simulink library "RWSW"  (Simulink 9.2)
settings: Solver=ode45  StartTime=0.0  StopTime=10.0  RelTol=1e-3  EnableMultiTasking=on
libraries: ACT x1, DYN x1, SEN x1
settings Model: Creator=alger  LastModifiedBy=alger

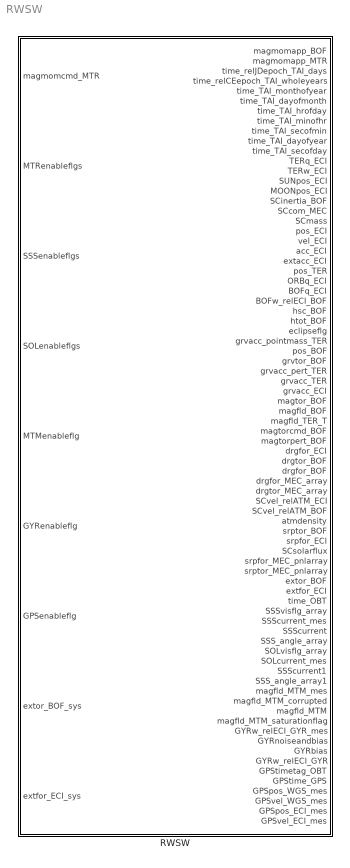
== system RWSW ==
  RWSW : Subsystem

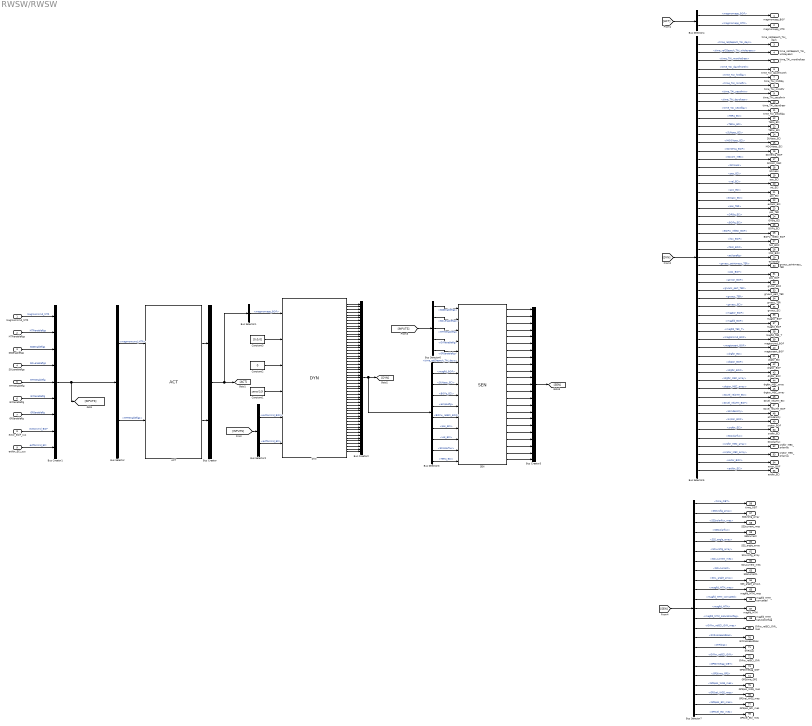
== system RWSW/RWSW ==
  magmomcmd_MTR : Inport  PortDimensions=10
  MTRenableflgs : Inport  Port=2  PortDimensions=10
  SSSenableflgs : Inport  Port=3  PortDimensions=10
  SOLenableflgs : Inport  Port=4  PortDimensions=10
  MTMenableflg : Inport  Port=5  PortDimensions=1
  GYRenableflg : Inport  Port=6  PortDimensions=1
  GPSenableflg : Inport  Port=7  PortDimensions=1
  extor_BOF_sys : Inport  Port=8  PortDimensions=3
  extfor_ECI_sys : Inport  Port=9  PortDimensions=3
  ACT : ACT/ACT  SystemSampleTime=-1
  Bus Creator : BusCreator  Inputs=2
  Bus Creator1 : BusCreator  Inputs=9
  Bus Creator2 : BusCreator  Inputs=55
  Bus Creator3 : BusCreator  Inputs=23
  Bus Selector : BusSelector  OutputSignals=magmomcmd_MTR,MTRenableflgs
  Bus Selector1 : BusSelector  OutputSignals=magmomapp_BOF
  Bus Selector2 : BusSelector  OutputSignals=exttorcmd_BOF,extforcmd_ECI
  Bus Selector3 : BusSelector  OutputSignals=time_relJDepoch_TAI_days,magfld_BOF,SUNpos_ECI,BOFq_ECI,eclipseflg,BOFw_relECI_BOF,pos_ECI,vel_ECI,SCsolarflux,TERq_ECI
  Bus Selector4 : BusSelector  OutputSignals=magmomapp_BOF,magmomapp_MTR
  Bus Selector5 : BusSelector  OutputSignals=time_relJDepoch_TAI_days,time_relCEepoch_TAI_wholeyears,time_TAI_monthofyear,time_TAI_dayofmonth,time_TAI_hrofday,time_TAI_minofhr,time_TAI_secofmin,time_TAI_dayofyear,time_TAI_secofday,TERq_ECI,TERw_ECI,SUNpos_ECI,MOONpos_ECI,SCinertia_BOF,SCcom_MEC,SCmass,pos_ECI,vel_ECI,acc_ECI,extacc_ECI,pos_TER,ORBq_ECI,BOFq_ECI,BOFw_relECI_BOF,hsc_BOF,htot_BOF,eclipseflg,grvacc_pointmass_TER,pos_BOF,grvtor_BOF,grvacc_pert_TER,grvacc_TER,grvacc_ECI,magtor_BOF,magfld_BOF,magfld_TER_T,magtorcmd_BOF,magtorpert_BOF,drgfor_ECI,drgtor_BOF,drgfor_BOF,drgfor_MEC_array,drgtor_MEC_array,SCvel_relATM_ECI,SCvel_relATM_BOF,atmdensity,srptor_BOF,srpfor_ECI,SCsolarflux,srpfor_MEC_array,srptor_MEC_array,extor_BOF,extfor_ECI
  Bus Selector6 : BusSelector  OutputSignals=SSSenableflgs,SOLenableflgs,MTMenableflg,GYRenableflg,GPSenableflg
  Bus Selector7 : BusSelector  OutputSignals=time_OBT,SSSvisflg_array,SSSsolarflux_mes,SSSsolarflux,SSS_angle_array,SOLvisflg_array,SOLcurrent_mes,SOLcurrent,SOL_angle_array,magfld_MTM_mes,magfld_MTM_corrupted,magfld_MTM,magfld_MTM_saturationflag,GYRw_relECI_GYR_mes,GYRnoiseandbias,GYRbias,GYRw_relECI_GYR,GPStimetag_OBT,GPStime_GPS,GPSpos_WGS_mes,GPSvel_WGS_mes,GPSpos_ECI_mes,GPSvel_ECI_mes
  Constant1 : Constant  Value=zeros(3,3)
  Constant2 : Constant  Value=0
  Constant3 : Constant  Value=[0;0;0]
  DYN : DYN/DYN  SystemSampleTime=-1
  SEN : SEN/SEN  SystemSampleTime=-1
  "magmomapp_BOF " : Outport
  magmomapp_MTR : Outport  Port=2
  time_relJDepoch_TAI_days : Outport  Port=3
  time_relCEepoch_TAI_wholeyears : Outport  Port=4
  time_TAI_monthofyear : Outport  Port=5
  time_TAI_dayofmonth : Outport  Port=6
  time_TAI_hrofday : Outport  Port=7
  time_TAI_minofhr : Outport  Port=8
  time_TAI_secofmin : Outport  Port=9
  time_TAI_dayofyear : Outport  Port=10
  time_TAI_secofday : Outport  Port=11
  TERq_ECI : Outport  Port=12
  TERw_ECI : Outport  Port=13
  SUNpos_ECI : Outport  Port=14
  MOONpos_ECI : Outport  Port=15
  SCinertia_BOF : Outport  Port=16
  SCcom_MEC : Outport  Port=17
  SCmass : Outport  Port=18
  pos_ECI : Outport  Port=19
  vel_ECI : Outport  Port=20
  acc_ECI : Outport  Port=21
  extacc_ECI : Outport  Port=22
  pos_TER : Outport  Port=23
  ORBq_ECI : Outport  Port=24
  BOFq_ECI : Outport  Port=25
  BOFw_relECI_BOF : Outport  Port=26
  hsc_BOF : Outport  Port=27
  htot_BOF : Outport  Port=28
  eclipseflg : Outport  Port=29
  grvacc_pointmass_TER : Outport  Port=30
  pos_BOF : Outport  Port=31
  grvtor_BOF : Outport  Port=32
  grvacc_pert_TER : Outport  Port=33
  grvacc_TER : Outport  Port=34
  grvacc_ECI : Outport  Port=35
  magtor_BOF : Outport  Port=36
  magfld_BOF : Outport  Port=37
  magfld_TER_T : Outport  Port=38
  magtorcmd_BOF : Outport  Port=39
  magtorpert_BOF : Outport  Port=40
  drgfor_ECI : Outport  Port=41
  drgtor_BOF : Outport  Port=42
  drgfor_BOF : Outport  Port=43
  drgfor_MEC_array : Outport  Port=44
  drgtor_MEC_array : Outport  Port=45
  SCvel_relATM_ECI : Outport  Port=46
  SCvel_relATM_BOF : Outport  Port=47
  atmdensity : Outport  Port=48
  srptor_BOF : Outport  Port=49  PortDimensions=3
  srpfor_ECI : Outport  Port=50  PortDimensions=3
  SCsolarflux : Outport  Port=51
  srpfor_MEC_pnlarray : Outport  Port=52
  srptor_MEC_pnlarray : Outport  Port=53
  extor_BOF : Outport  Port=54
  extfor_ECI : Outport  Port=55
  time_OBT : Outport  Port=56
  SSSvisflg_array : Outport  Port=57
  SSScurrent_mes : Outport  Port=58
  SSScurrent : Outport  Port=59
  SSS_angle_array : Outport  Port=60
  SOLvisflg_array : Outport  Port=61
  SOLcurrent_mes : Outport  Port=62
  SSScurrent1 : Outport  Port=63
  SSS_angle_array1 : Outport  Port=64
  magfld_MTM_mes : Outport  Port=65
  magfld_MTM_corrupted : Outport  Port=66
  magfld_MTM : Outport  Port=67
  magfld_MTM_saturationflag : Outport  Port=68
  GYRw_relECI_GYR_mes : Outport  Port=69  PortDimensions=3
  GYRnoiseandbias : Outport  Port=70  PortDimensions=3
  GYRbias : Outport  Port=71  PortDimensions=3
  GYRw_relECI_GYR : Outport  Port=72  PortDimensions=3
  GPStimetag_OBT : Outport  Port=73
  GPStime_GPS : Outport  Port=74
  GPSpos_WGS_mes : Outport  Port=75
  GPSvel_WGS_mes : Outport  Port=76
  GPSpos_ECI_mes : Outport  Port=77
  GPSvel_ECI_mes : Outport  Port=78
  wires:
  magmomcmd_MTR/1 -> Bus Creator1/1  "magmomcmd_MTR"
  Constant1/1 -> DYN/4
  ACT/1 -> Bus Creator/1
  ACT/2 -> Bus Creator/2
  extor_BOF_sys/1 -> Bus Creator1/8  "exttorcmd_BOF"
  extfor_ECI_sys/1 -> Bus Creator1/9  "extforcmd_ECI"
  Bus Creator1/1 -> Bus Selector/1, [INPUTS]
  Bus Selector/1 -> ACT/1  "<magmomcmd_MTR>"
  Bus Creator/1 -> Bus Selector1/1, [ACT]
  Constant2/1 -> DYN/3
  Constant3/1 -> DYN/2
  Bus Selector1/1 -> DYN/1  "<magmomapp_BOF>"
  [INPUTS] -> Bus Selector2/1
  Bus Selector2/1 -> DYN/5  "<exttorcmd_BOF>"
  Bus Selector2/2 -> DYN/6  "<extforcmd_ECI>"
  DYN/31 -> Bus Creator2/31
  DYN/10 -> Bus Creator2/10
  DYN/23 -> Bus Creator2/23
  DYN/27 -> Bus Creator2/27
  DYN/3 -> Bus Creator2/3
  DYN/46 -> Bus Creator2/46
  DYN/47 -> Bus Creator2/47
  DYN/22 -> Bus Creator2/22
  DYN/35 -> Bus Creator2/35
  DYN/37 -> Bus Creator2/37
  DYN/36 -> Bus Creator2/36
  DYN/2 -> Bus Creator2/2
  DYN/38 -> Bus Creator2/38
  DYN/40 -> Bus Creator2/40
  DYN/12 -> Bus Creator2/12
  DYN/24 -> Bus Creator2/24
  DYN/11 -> Bus Creator2/11
  DYN/42 -> Bus Creator2/42
  DYN/48 -> Bus Creator2/48
  DYN/26 -> Bus Creator2/26
  DYN/5 -> Bus Creator2/5
  DYN/8 -> Bus Creator2/8
  DYN/7 -> Bus Creator2/7
  DYN/13 -> Bus Creator2/13
  DYN/14 -> Bus Creator2/14
  DYN/16 -> Bus Creator2/16
  DYN/34 -> Bus Creator2/34
  DYN/41 -> Bus Creator2/41
  DYN/43 -> Bus Creator2/43
  DYN/6 -> Bus Creator2/6
  DYN/15 -> Bus Creator2/15
  DYN/49 -> Bus Creator2/49
  DYN/9 -> Bus Creator2/9
  DYN/50 -> Bus Creator2/50
  DYN/19 -> Bus Creator2/19
  DYN/4 -> Bus Creator2/4
  DYN/1 -> Bus Creator2/1
  DYN/18 -> Bus Creator2/18
  DYN/25 -> Bus Creator2/25
  DYN/29 -> Bus Creator2/29
  DYN/30 -> Bus Creator2/30
  DYN/20 -> Bus Creator2/20
  DYN/32 -> Bus Creator2/32
  DYN/28 -> Bus Creator2/28
  DYN/52 -> Bus Creator2/52
  DYN/21 -> Bus Creator2/21
  DYN/33 -> Bus Creator2/33
  DYN/39 -> Bus Creator2/39
  DYN/53 -> Bus Creator2/53
  DYN/17 -> Bus Creator2/17
  DYN/51 -> Bus Creator2/51
  DYN/44 -> Bus Creator2/44
  DYN/45 -> Bus Creator2/45
  Bus Creator2/1 -> Bus Selector3/1, [DYN]
  [ACT] -> Bus Selector4/1
  Bus Selector4/1 -> "magmomapp_BOF "/1  "<magmomapp_BOF>"
  Bus Selector4/2 -> magmomapp_MTR/1  "<magmomapp_MTR>"
  [DYN] -> Bus Selector5/1
  Bus Selector5/10 -> TERq_ECI/1  "<TERq_ECI>"
  Bus Selector5/11 -> TERw_ECI/1  "<TERw_ECI>"
  Bus Selector5/13 -> MOONpos_ECI/1  "<MOONpos_ECI>"
  Bus Selector5/12 -> SUNpos_ECI/1  "<SUNpos_ECI>"
  Bus Selector5/16 -> SCmass/1  "<SCmass>"
  Bus Selector5/15 -> SCcom_MEC/1  "<SCcom_MEC>"
  Bus Selector5/14 -> SCinertia_BOF/1  "<SCinertia_BOF>"
  Bus Selector5/22 -> ORBq_ECI/1  "<ORBq_ECI>"
  Bus Selector5/21 -> pos_TER/1  "<pos_TER>"
  Bus Selector5/19 -> acc_ECI/1  "<acc_ECI>"
  Bus Selector5/18 -> vel_ECI/1  "<vel_ECI>"
  Bus Selector5/17 -> pos_ECI/1  "<pos_ECI>"
  Bus Selector5/20 -> extacc_ECI/1  "<extacc_ECI>"
  Bus Selector5/2 -> time_relCEepoch_TAI_wholeyears/1  "<time_relCEepoch_TAI_wholeyears>"
  Bus Selector5/3 -> time_TAI_monthofyear/1  "<time_TAI_monthofyear>"
  Bus Selector5/6 -> time_TAI_minofhr/1  "<time_TAI_minofhr>"
  Bus Selector5/9 -> time_TAI_secofday/1  "<time_TAI_secofday>"
  Bus Selector5/1 -> time_relJDepoch_TAI_days/1  "<time_relJDepoch_TAI_days>"
  Bus Selector5/7 -> time_TAI_secofmin/1  "<time_TAI_secofmin>"
  Bus Selector5/4 -> time_TAI_dayofmonth/1  "<time_TAI_dayofmonth>"
  Bus Selector5/5 -> time_TAI_hrofday/1  "<time_TAI_hrofday>"
  Bus Selector5/8 -> time_TAI_dayofyear/1  "<time_TAI_dayofyear>"
  Bus Selector5/23 -> BOFq_ECI/1  "<BOFq_ECI>"
  Bus Selector5/24 -> BOFw_relECI_BOF/1  "<BOFw_relECI_BOF>"
  Bus Selector5/25 -> hsc_BOF/1  "<hsc_BOF>"
  Bus Selector5/26 -> htot_BOF/1  "<htot_BOF>"
  Bus Selector5/27 -> eclipseflg/1  "<eclipseflg>"
  Bus Selector5/28 -> grvacc_pointmass_TER/1  "<grvacc_pointmass_TER>"
  Bus Selector5/29 -> pos_BOF/1  "<pos_BOF>"
  Bus Selector5/30 -> grvtor_BOF/1  "<grvtor_BOF>"
  Bus Selector5/31 -> grvacc_pert_TER/1  "<grvacc_pert_TER>"
  Bus Selector5/32 -> grvacc_TER/1  "<grvacc_TER>"
  Bus Selector5/33 -> grvacc_ECI/1  "<grvacc_ECI>"
  Bus Selector5/34 -> magtor_BOF/1  "<magtor_BOF>"
  Bus Selector5/36 -> magfld_TER_T/1  "<magfld_TER_T>"
  Bus Selector5/38 -> magtorpert_BOF/1  "<magtorpert_BOF>"
  Bus Selector5/35 -> magfld_BOF/1  "<magfld_BOF>"
  Bus Selector5/37 -> magtorcmd_BOF/1  "<magtorcmd_BOF>"
  Bus Selector5/44 -> SCvel_relATM_ECI/1  "<SCvel_relATM_ECI>"
  Bus Selector5/39 -> drgfor_ECI/1  "<drgfor_ECI>"
  Bus Selector5/42 -> drgfor_MEC_array/1  "<drgfor_MEC_array>"
  Bus Selector5/43 -> drgtor_MEC_array/1  "<drgtor_MEC_array>"
  Bus Selector5/45 -> SCvel_relATM_BOF/1  "<SCvel_relATM_BOF>"
  Bus Selector5/46 -> atmdensity/1  "<atmdensity>"
  Bus Selector5/40 -> drgtor_BOF/1  "<drgtor_BOF>"
  Bus Selector5/41 -> drgfor_BOF/1  "<drgfor_BOF>"
  Bus Selector5/47 -> srptor_BOF/1  "<srptor_BOF>"
  Bus Selector5/48 -> srpfor_ECI/1  "<srpfor_ECI>"
  Bus Selector5/49 -> SCsolarflux/1  "<SCsolarflux>"
  Bus Selector5/50 -> srpfor_MEC_pnlarray/1  "<srpfor_MEC_array>"
  Bus Selector5/51 -> srptor_MEC_pnlarray/1  "<srptor_MEC_array>"
  Bus Selector5/52 -> extor_BOF/1  "<extor_BOF>"
  Bus Selector5/53 -> extfor_ECI/1  "<extfor_ECI>"
  MTRenableflgs/1 -> Bus Creator1/2  "MTRenableflgs"
  Bus Selector/2 -> ACT/2  "<MTRenableflgs>"
  [INPUTS] -> Bus Selector6/1
  MTMenableflg/1 -> Bus Creator1/5  "MTMenableflg"
  SSSenableflgs/1 -> Bus Creator1/3  "SSSenableflgs"
  GYRenableflg/1 -> Bus Creator1/6  "GYRenableflg"
  GPSenableflg/1 -> Bus Creator1/7  "GPSenableflg"
  Bus Creator3/1 -> [SEN]
  [SEN] -> Bus Selector7/1
  SOLenableflgs/1 -> Bus Creator1/4  "SOLenableflgs"
  Bus Selector6/2 -> SEN/2  "<SOLenableflgs>"
  Bus Selector6/4 -> SEN/4  "<GYRenableflg>"
  Bus Selector6/1 -> SEN/1  "<SSSenableflgs>"
  Bus Selector6/3 -> SEN/3  "<MTMenableflg>"
  Bus Selector6/5 -> SEN/5  "<GPSenableflg>"
  Bus Selector3/6 -> SEN/11  "<BOFw_relECI_BOF>"
  Bus Selector3/5 -> SEN/10  "<eclipseflg>"
  Bus Selector3/7 -> SEN/12  "<pos_ECI>"
  Bus Selector3/4 -> SEN/9  "<BOFq_ECI>"
  Bus Selector3/8 -> SEN/13  "<vel_ECI>"
  Bus Selector3/9 -> SEN/14  "<SCsolarflux>"
  Bus Selector3/3 -> SEN/8  "<SUNpos_ECI>"
  Bus Selector3/2 -> SEN/7  "<magfld_BOF>"
  Bus Selector3/1 -> SEN/6  "<time_relJDepoch_TAI_days>"
  SEN/1 -> Bus Creator3/1
  SEN/5 -> Bus Creator3/5
  SEN/17 -> Bus Creator3/17
  SEN/18 -> Bus Creator3/18
  SEN/20 -> Bus Creator3/20
  SEN/21 -> Bus Creator3/21
  SEN/22 -> Bus Creator3/22
  SEN/4 -> Bus Creator3/4
  SEN/8 -> Bus Creator3/8
  SEN/10 -> Bus Creator3/10
  SEN/19 -> Bus Creator3/19
  SEN/9 -> Bus Creator3/9
  SEN/11 -> Bus Creator3/11
  SEN/2 -> Bus Creator3/2
  SEN/12 -> Bus Creator3/12
  SEN/6 -> Bus Creator3/6
  SEN/15 -> Bus Creator3/15
  SEN/13 -> Bus Creator3/13
  SEN/7 -> Bus Creator3/7
  SEN/3 -> Bus Creator3/3
  SEN/14 -> Bus Creator3/14
  SEN/16 -> Bus Creator3/16
  Bus Selector7/1 -> time_OBT/1  "<time_OBT>"
  Bus Selector7/2 -> SSSvisflg_array/1  "<SSSvisflg_array>"
  Bus Selector7/3 -> SSScurrent_mes/1  "<SSSsolarflux_mes>"
  Bus Selector7/4 -> SSScurrent/1  "<SSSsolarflux>"
  Bus Selector7/5 -> SSS_angle_array/1  "<SSS_angle_array>"
  Bus Selector7/6 -> SOLvisflg_array/1  "<SOLvisflg_array>"
  Bus Selector7/7 -> SOLcurrent_mes/1  "<SOLcurrent_mes>"
  Bus Selector7/8 -> SSScurrent1/1  "<SOLcurrent>"
  Bus Selector7/9 -> SSS_angle_array1/1  "<SOL_angle_array>"
  Bus Selector7/10 -> magfld_MTM_mes/1  "<magfld_MTM_mes>"
  Bus Selector7/11 -> magfld_MTM_corrupted/1  "<magfld_MTM_corrupted>"
  Bus Selector7/12 -> magfld_MTM/1  "<magfld_MTM>"
  Bus Selector7/18 -> GPStimetag_OBT/1  "<GPStimetag_OBT>"
  Bus Selector7/15 -> GYRnoiseandbias/1  "<GYRnoiseandbias>"
  Bus Selector7/19 -> GPStime_GPS/1  "<GPStime_GPS>"
  Bus Selector7/17 -> GYRw_relECI_GYR/1  "<GYRw_relECI_GYR>"
  Bus Selector7/14 -> GYRw_relECI_GYR_mes/1  "<GYRw_relECI_GYR_mes>"
  Bus Selector7/16 -> GYRbias/1  "<GYRbias>"
  Bus Selector7/21 -> GPSvel_WGS_mes/1  "<GPSvel_WGS_mes>"
  Bus Selector7/22 -> GPSpos_ECI_mes/1  "<GPSpos_ECI_mes>"
  Bus Selector7/23 -> GPSvel_ECI_mes/1  "<GPSvel_ECI_mes>"
  Bus Selector7/20 -> GPSpos_WGS_mes/1  "<GPSpos_WGS_mes>"
  SEN/23 -> Bus Creator3/23
  Bus Selector7/13 -> magfld_MTM_saturationflag/1  "<magfld_MTM_saturationflag>"
  DYN/54 -> Bus Creator2/54
  DYN/55 -> Bus Creator2/55
  Bus Selector3/10 -> SEN/15  "<TERq_ECI>"
